simulink model "CU_Basico_Masetti"  (R2018a)
settings: Solver=FixedStepAuto  StartTime=0.0  StopTime=0.005  RelTol=1e-3
values from neighbouring files (symbols this model uses):
  Fincognita = 25000    [Init.m]
  Fr = 1000000    [Init.m]
libraries: powerlib_meascontrol x2, simulink_extras x1, dspswit3 x1
settings Model: Creator=Augusto  LastModifiedBy=Augusto

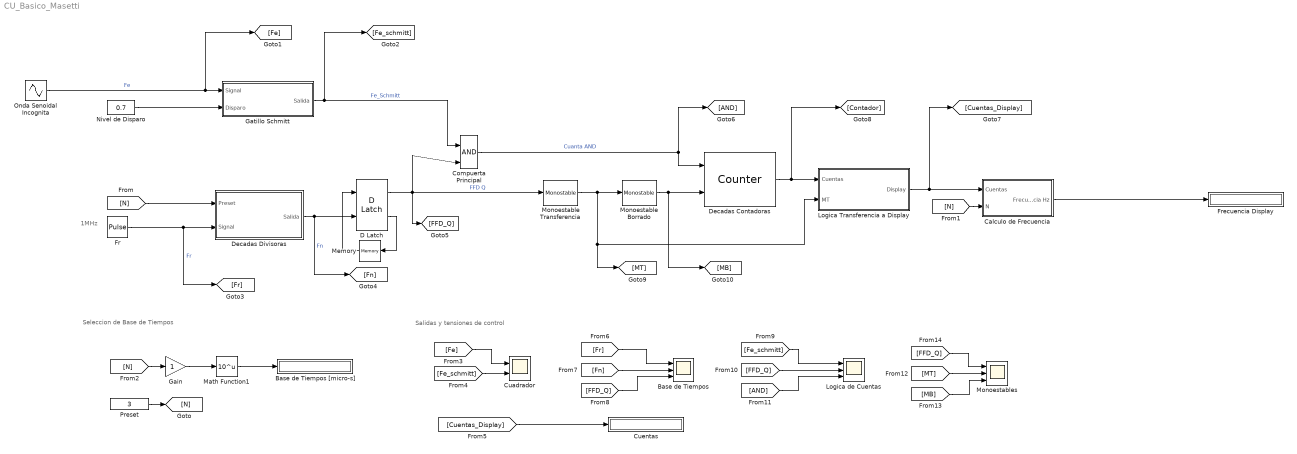
== system CU_Basico_Masetti ==
  note: Salidas y tensiones de control
  note: Seleccion de Base de Tiempos
  note: 1MHz
  Base de Tiempos : Scope  NumInputPorts=3
  Base de Tiempos [micro-s] : Display
  Calculo de Frecuencia : Subsystem
  Compuerta Principal : Logic  IconShape=distinctive  AllPortsSameDT=off  OutDataTypeStr=boolean
  Cuadrador : Scope  NumInputPorts=2
  Cuentas : Display
  D Latch : simulink_extras/Flip Flops/D Latch
      settings: SourceProductName=Simulink  SourceProductBaseCode=SL
  Decadas Contadoras : dspswit3/Counter  Direction=Up  CountEvent=Rising edge  CounterSize=User defined  MaxCount=1000  InitialCount=0  Output=Count  HitValue=32  ResetInput=on  SamplesPerFrame=1  Ts=1  CntDtype=double  HitDtype=Logical
  Decadas Divisoras : MATLAB Function  TreatAsAtomicUnit=on
  Fr : DiscretePulseGenerator  PulseType=Time based  Period=1/Fr  PulseWidth=50
  Frecuencia Display : Display
  Gain : Gain
  Gatillo Schmitt : MATLAB Function  TreatAsAtomicUnit=on
  Logica Transferencia a Display : MATLAB Function  TreatAsAtomicUnit=on
  Logica de Cuentas : Scope  NumInputPorts=3
  Math Function1 : Math  Operator=10^u  SaturateOnIntegerOverflow=on
  Memory : Memory  InheritSampleTime=on
  "Monoestable Borrado " : powerlib_meascontrol/Logic/Monostable  EdgeDetect=Falling  PulseDuration=0.5/Fr  ic=0  Ts=0
      settings: SourceProductName=Simscape Power Systems  SourceProductBaseCode=PS
  Monoestable Transferencia : powerlib_meascontrol/Logic/Monostable  EdgeDetect=Falling  PulseDuration=0.5/Fr  ic=0  Ts=0
      settings: SourceProductName=Simscape Power Systems  SourceProductBaseCode=PS
  Monoestables : Scope  NumInputPorts=3
  Nivel de Disparo : Constant  Value=0.7
  Onda Senoidal Incognita : Sin  Frequency=2*pi*Fincognita  SampleTime=0
  "Preset " : Constant  Value=3
  wires:
  D Latch/1 -> [FFD_Q], Monoestable Transferencia/1, Compuerta Principal/2  "FFD Q"
  Compuerta Principal/1 -> Decadas Contadoras/1, [AND]  "Cuanta AND"
  D Latch/2 -> Memory/1
  Memory/1 -> D Latch/1
  Monoestable Transferencia/1 -> [MT], Logica Transferencia a Display/2(MT), "Monoestable Borrado "/1
  "Monoestable Borrado "/1 -> [MB], Decadas Contadoras/2
  Decadas Contadoras/1 -> [Contador], Logica Transferencia a Display/1(Cuentas)
  Fr/1 -> [Fr], Decadas Divisoras/2(Signal)  "Fr"
  Onda Senoidal Incognita/1 -> [Fe], Gatillo Schmitt/1(Signal)  "Fe"
  Nivel de Disparo/1 -> Gatillo Schmitt/2(Disparo)
  Gatillo Schmitt/1(Salida) -> [Fe_schmitt], Compuerta Principal/1  "Fe_Schmitt"
  Decadas Divisoras/1(Salida) -> [Fn], D Latch/2  "Fn"
  "Preset "/1 -> [N]
  [N] -> Decadas Divisoras/1(Preset)
  Logica Transferencia a Display/1(Display) -> [Cuentas_Display], Calculo de Frecuencia/1(Cuentas)
  Math Function1/1 -> Base de Tiempos [micro-s]/1
  [N] -> Gain/1
  Gain/1 -> Math Function1/1
  [N] -> Calculo de Frecuencia/2(N)
  Calculo de Frecuencia/1(Frecuencia Hz) -> Frecuencia Display/1
  [Cuentas_Display] -> Cuentas/1
  [FFD_Q] -> Monoestables/1
  [MT] -> Monoestables/2
  [MB] -> Monoestables/3
  [FFD_Q] -> Logica de Cuentas/2
  [Fe_schmitt] -> Logica de Cuentas/1
  [AND] -> Logica de Cuentas/3
  [Fn] -> Base de Tiempos/2
  [FFD_Q] -> Base de Tiempos/3
  [Fr] -> Base de Tiempos/1
  [Fe] -> Cuadrador/1
  [Fe_schmitt] -> Cuadrador/2

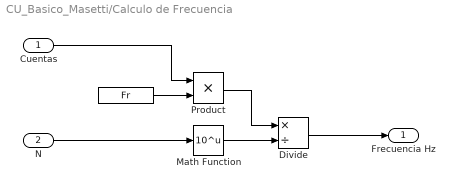
== system CU_Basico_Masetti/Calculo de Frecuencia ==
  Cuentas : Inport
  N : Inport  Port=2
  " " : Constant  Value=Fr
  Divide : Product  Inputs=*/
  Math Function : Math  Operator=10^u  SaturateOnIntegerOverflow=on
  Product : Product
  Frecuencia Hz : Outport
  wires:
  Product/1 -> Divide/1
  Divide/1 -> Frecuencia Hz/1
  Math Function/1 -> Divide/2
  " "/1 -> Product/2
  N/1 -> Math Function/1
  Cuentas/1 -> Product/1

== matlab function CU_Basico_Masetti/Decadas Divisoras ==
  data: Preset input; Signal input; Salida output
function Salida = fcn(Preset,Signal)
    persistent count 
    persistent ant
    if isempty(ant)
        ant=0;
    end
    if isempty(count)
        count=0;
    end
    if count == 0 && Signal ==1 
        Salida = 1;
    else
        Salida = 0;
    end
    if ant ~= Signal
        count = count + 1;
    end
    if count == 10^Preset
        count = 0;
    end

== matlab function CU_Basico_Masetti/Gatillo Schmitt ==
  data: Signal input; Salida output; Disparo input
function Salida = fcn(Signal,Disparo)
     
    persistent u 
    if isempty(u)
        u=0;
    else
        if(Signal<=-Disparo) 
            u = 0;
        end
        if(Signal>Disparo)
            u = 1;
        end
    end
    
    Salida = u;

== matlab function CU_Basico_Masetti/Logica Transferencia a Display ==
  data: Cuentas input; MT input; Display output
function Display = fcn(Cuentas,MT)
    persistent display 
    if isempty(display)
        display=0;
    end

    if MT ==1  
        display = Cuentas;
    end
    Display = display;
